simulink model "Iac"  (R2021a)
settings: Solver=ode45  StartTime=0.0  StopTime=10.0  RelTol=1e-3  EnableMultiTasking=on
undefined symbols (not defined in the file): Iac_degIgnOptOffset, Iac_flgIgnCutoffReq, Iac_pManiReqMin, sample_z
libraries: simulink x1
settings Model: Creator=YAL9FE  LastModifiedBy=FPR9FE
settings SolverCC: AlgebraicLoopSolver=TrustRegion
settings DataIOCC: LimitDataPoints=on  SaveFormat=Array  SignalLoggingSaveFormat=ModelDataLogs  ReturnWorkspaceOutputs=off
settings OptimizationCC: ExpressionDepthLimit=2147483647  LifeSpan=inf
settings DebuggingCC: UnderspecifiedInitializationDetection=Classic  MergeDetectMultiDrivingBlocksExec=none  SolverPrmCheckMsg=warning  FcnCallInpInsideContextMsg=warning  StateNameClashWarn=warning  SFUnexpectedBacktrackingDiag=warning  SFNoUnconditionalDefaultTransitionDiag=warning  SFExecutionAtInitializationDiag=none  SFMachineParentedDataDiag=warning  ArithmeticOperatorsInVariantConditions=warning
settings HardwareCC: ProdBitPerPointer=32  ProdBitPerSizeT=32  ProdBitPerPtrDiffT=32  ProdLargestAtomicFloat=None  ProdIntDivRoundTo=Undefined  ProdEndianess=Unspecified  ProdWordSize=32  ProdHWDeviceType=32-bit Generic
settings ModelReferenceCC: PropagateSignalLabelsOutOfModel=off
settings SFSimCC: SimUseLocalCustomCode=off  CustomCodeUndefinedFunction=UseInterfaceOnly
settings RTWCC: RTWUseLocalCustomCode=off
settings CodeAppCC: StateflowObjectComments=on
settings GRTTargetCC: TargetLangStandard=C89/C90 (ANSI)  CombineOutputUpdateFcns=off  GRTInterface=on
settings ConfigComp: CovMetricSettings=dw  CovSaveCumulativeToWorkspaceVar=on  CovSaveSingleToWorkspaceVar=on  CovExternalEMLEnable=off  CovSFcnEnable=off

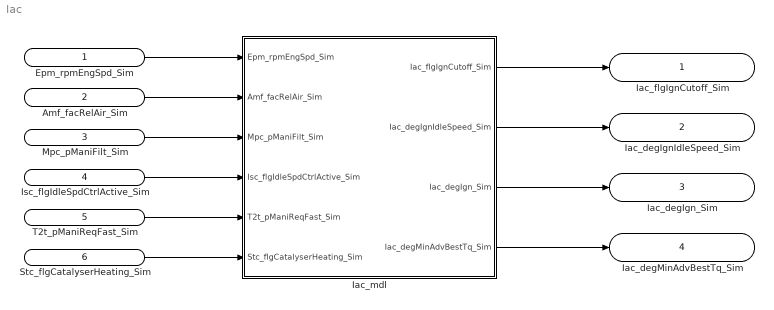
== system Iac ==
  Epm_rpmEngSpd_Sim : Inport
  Amf_facRelAir_Sim : Inport  Port=2
  Mpc_pManiFilt_Sim : Inport  Port=3
  Isc_flgIdleSpdCtrlActive_Sim : Inport  Port=4
  T2t_pManiReqFast_Sim : Inport  Port=5
  Stc_flgCatalyserHeating_Sim : Inport  Port=6
  Iac_mdl : Subsystem  mask(Functions){}
      mask help: IgnitionAngle
      mask Display:
      | image(imread('IgnitionAngle.jpg'))
      | port_label('input',1,'Epm_rpmEngSpd_Sim')
      | port_label('input',2,'Amf_facRelAir_Sim')
      | port_label('input',3,'Mpc_pManiFilt_Sim')
      | port_label('input',4,'Isc_flgIdleSpdCtrlActive_Sim')
      | port_label('input',5,'T2t_pManiReqFast_Sim')
      | port_label('input',6,'Stc_flgCatalyserHeating_Sim')
      | port_label('output',1,'Iac_flgIgnCutoff_Sim')
      | port_label('output',2,'Iac_degIgnIdleSpeed_Sim')
      | port_label('output',3,'Iac_degIgn_Sim')
      | port_label('output',4,'Iac_degMinAdvBestTq_Sim')
  Iac_flgIgnCutoff_Sim : Outport
  Iac_degIgnIdleSpeed_Sim : Outport  Port=2
  Iac_degIgn_Sim : Outport  Port=3
  Iac_degMinAdvBestTq_Sim : Outport  Port=4
  wires:
  Epm_rpmEngSpd_Sim/1 -> Iac_mdl/1(Epm_rpmEngSpd_Sim)
  Amf_facRelAir_Sim/1 -> Iac_mdl/2(Amf_facRelAir_Sim)
  Mpc_pManiFilt_Sim/1 -> Iac_mdl/3(Mpc_pManiFilt_Sim)
  Isc_flgIdleSpdCtrlActive_Sim/1 -> Iac_mdl/4(Isc_flgIdleSpdCtrlActive_Sim)
  T2t_pManiReqFast_Sim/1 -> Iac_mdl/5(T2t_pManiReqFast_Sim)
  Iac_mdl/1(Iac_flgIgnCutoff_Sim) -> Iac_flgIgnCutoff_Sim/1
  Iac_mdl/2(Iac_degIgnIdleSpeed_Sim) -> Iac_degIgnIdleSpeed_Sim/1
  Iac_mdl/3(Iac_degIgn_Sim) -> Iac_degIgn_Sim/1
  Iac_mdl/4(Iac_degMinAdvBestTq_Sim) -> Iac_degMinAdvBestTq_Sim/1
  Stc_flgCatalyserHeating_Sim/1 -> Iac_mdl/6(Stc_flgCatalyserHeating_Sim)

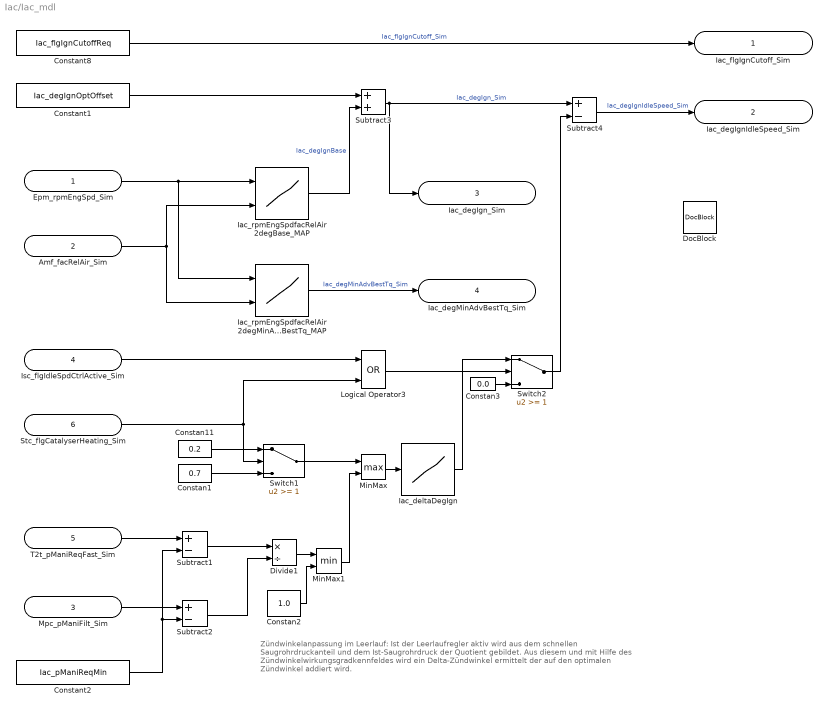
== system Iac/Iac_mdl ==
  note: Zündwinkelanpassung im Leerlauf:
      | Ist der Leerlaufregler aktiv wird aus dem schnellen Saugrohrdruckanteil und dem Ist-Saugrohrdruck
      | der Quotient gebildet. Aus diesem und mit Hilfe des Zündwinkelwirkungsgradkennfeldes wird ein
      | Delta-Zündwinkel ermittelt der auf den optimalen Zündwinkel addiert wird.
  Epm_rpmEngSpd_Sim : Inport
  Amf_facRelAir_Sim : Inport  Port=2
  Mpc_pManiFilt_Sim : Inport  Port=3
  Isc_flgIdleSpdCtrlActive_Sim : Inport  Port=4
  T2t_pManiReqFast_Sim : Inport  Port=5
  Stc_flgCatalyserHeating_Sim : Inport  Port=6
  Constan1 : Constant  Value=0.7  OutDataTypeStr=single
  Constan11 : Constant  Value=0.2  OutDataTypeStr=single
  Constan2 : Constant  Value=1.0  OutDataTypeStr=single
  Constan3 : Constant  Value=0.0  OutDataTypeStr=single
  Constant1 : Constant  Value=Iac_degIgnOptOffset
  Constant2 : Constant  Value=Iac_pManiReqMin
  Constant8 : Constant  Value=Iac_flgIgnCutoffReq
  Divide1 : Product  Inputs=*/  OutDataTypeStr=Inherit: Same as first input
  DocBlock : simulink/Model-Wide Utilities/DocBlock  DocumentType=Text
      content=|
      | In the IgnitionAngle module, the base ignition angle Iac_degIgnBase and the optimum ignition angle Iac_degMinAdvBestTq_Sim are determined from the speed Epm_rpmEngSpd_Sim and the re- lative fill Amf_facRelAir_Sim. The base ignition angle describes the angle of the highest torque at which just no knocking occurs. It is calculated via the map Iac_rpmEngSpdfacRelAir2degBase_MAP and can then be shifted late with the offset Iac_degIgnOptOffset for safety before the ignition angle to be set Iac_degIgn_Sim is passed on as a message. In contrast to smart engine control, a positive value means that ignition takes place before the upper ignition dead center, and a negative angle after it, i.e. the ignition angle is pulled late by the basic parameterization of the offset Iac_degIgnOptOffset with -5.0°KW.
  Iac_deltaDegIgn : Lookup_n-D  NumberOfTableDimensions=1  BreakpointsForDimension1=[1:3]  Table=[10 18 23]  ExtrapMethod=Clip  InputSameDT=on
      settings: AttributesFormatString=%<Table>
  Iac_rpmEngSpdfacRelAir2degBase_MAP : Lookup_n-D  BreakpointsForDimension1=[1:3]  BreakpointsForDimension2=[1:3]  Table=sample_z  ExtrapMethod=Clip  InputSameDT=on
      settings: AttributesFormatString=%<Table>  InputPortMap=u0,u1
  Iac_rpmEngSpdfacRelAir2degMinAdvBestTq_MAP : Lookup_n-D  BreakpointsForDimension1=[1:3]  BreakpointsForDimension2=[1:3]  ExtrapMethod=Clip  InputSameDT=on
      settings: AttributesFormatString=%<Table>  InputPortMap=u0,u1
  Logical Operator3 : Logic  Operator=OR  AllPortsSameDT=off  OutDataTypeStr=boolean
  MinMax : MinMax  Function=max  Inputs=2
  MinMax1 : MinMax  Inputs=2
  Subtract1 : Sum  Inputs=+-  OutDataTypeStr=Inherit: Same as first input
  Subtract2 : Sum  Inputs=+-  OutDataTypeStr=Inherit: Same as first input
  Subtract3 : Sum  OutDataTypeStr=Inherit: Same as first input
  Subtract4 : Sum  Inputs=+-  OutDataTypeStr=Inherit: Same as first input
  Switch1 : Switch  Threshold=1
  Switch2 : Switch  Threshold=1
  Iac_flgIgnCutoff_Sim : Outport
  Iac_degIgnIdleSpeed_Sim : Outport  Port=2
  Iac_degIgn_Sim : Outport  Port=3
  Iac_degMinAdvBestTq_Sim : Outport  Port=4
  wires:
  Constant8/1 -> Iac_flgIgnCutoff_Sim/1  "Iac_flgIgnCutoff_Sim"
  Constant1/1 -> Subtract3/1
  Iac_rpmEngSpdfacRelAir2degBase_MAP/1 -> Subtract3/2  "Iac_degIgnBase"
  Epm_rpmEngSpd_Sim/1 -> Iac_rpmEngSpdfacRelAir2degBase_MAP/1, Iac_rpmEngSpdfacRelAir2degMinAdvBestTq_MAP/1
  Amf_facRelAir_Sim/1 -> Iac_rpmEngSpdfacRelAir2degBase_MAP/2, Iac_rpmEngSpdfacRelAir2degMinAdvBestTq_MAP/2
  Constan1/1 -> Switch1/3
  Stc_flgCatalyserHeating_Sim/1 -> Switch1/2, Logical Operator3/2
  Constan11/1 -> Switch1/1
  Switch1/1 -> MinMax/1
  T2t_pManiReqFast_Sim/1 -> Subtract1/1
  Subtract1/1 -> Divide1/1
  Constant2/1 -> Subtract1/2, Subtract2/2
  Mpc_pManiFilt_Sim/1 -> Subtract2/1
  Subtract2/1 -> Divide1/2
  MinMax1/1 -> MinMax/2
  Divide1/1 -> MinMax1/1
  Constan2/1 -> MinMax1/2
  Iac_rpmEngSpdfacRelAir2degMinAdvBestTq_MAP/1 -> Iac_degMinAdvBestTq_Sim/1  "Iac_degMinAdvBestTq_Sim"
  Subtract3/1 -> Iac_degIgn_Sim/1, Subtract4/1  "Iac_degIgn_Sim"
  Subtract4/1 -> Iac_degIgnIdleSpeed_Sim/1  "Iac_degIgnIdleSpeed_Sim"
  Isc_flgIdleSpdCtrlActive_Sim/1 -> Logical Operator3/1
  Logical Operator3/1 -> Switch2/2
  Switch2/1 -> Subtract4/2
  Iac_deltaDegIgn/1 -> Switch2/1
  Constan3/1 -> Switch2/3
  MinMax/1 -> Iac_deltaDegIgn/1
